simulink model "HinfController"  (R2024b)
settings: Solver=FixedStepDiscrete  StartTime=0.0  StopTime=Inf  FixedStep=0.001  RelTol=1e-3
model workspace (MAT data in the model file):
  robot : robotics.RigidBodyTree (value not decoded)
settings Model: Creator=sung  LastModifiedBy=sung
settings HardwareCC: ProdBitPerLong=64  ProdHWDeviceType=Intel->x86-64 (Linux 64)
settings RTWCC: GenCodeOnly=on  Toolchain=CMake

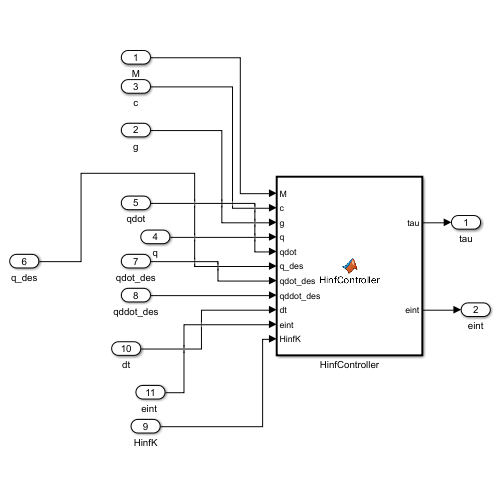
[thumbnail: Simulink's stored preview of the top-level diagram]
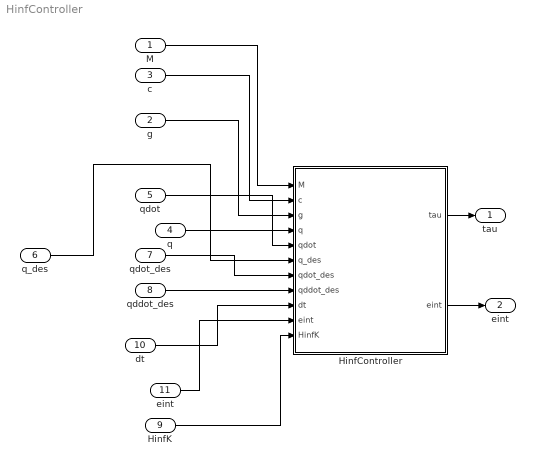
== system HinfController ==
  M : Inport  PortDimensions=[12,12]
  g : Inport  Port=2  PortDimensions=12
  c : Inport  Port=3  PortDimensions=12
  q : Inport  Port=4  PortDimensions=12
  qdot : Inport  Port=5  PortDimensions=12
  q_des : Inport  Port=6  PortDimensions=12
  qdot_des : Inport  Port=7  PortDimensions=12
  qddot_des : Inport  Port=8  PortDimensions=12
  HinfK : Inport  Port=9  PortDimensions=12
  dt : Inport  Port=10
  "eint " : Inport  Port=11
  HinfController : MATLAB Function  TreatAsAtomicUnit=on
  tau : Outport
  eint : Outport  Port=2
  wires:
  M/1 -> HinfController/1(M)
  qdot_des/1 -> HinfController/7(qdot_des)
  g/1 -> HinfController/3(g)
  c/1 -> HinfController/2(c)
  q/1 -> HinfController/4(q)
  qdot/1 -> HinfController/5(qdot)
  q_des/1 -> HinfController/6(q_des)
  qddot_des/1 -> HinfController/8(qddot_des)
  HinfController/1(tau) -> tau/1
  HinfController/2(eint) -> eint/1
  HinfK/1 -> HinfController/11(HinfK)
  dt/1 -> HinfController/9(dt)
  "eint "/1 -> HinfController/10("eint ")

== matlab function HinfController/HinfController ==
  data: M input size=[12,12]; tau output size=[12,1]; c input size=[12,1]; g input size=[12,1]; q input size=[12,1]; qdot input size=[12,1]; q_des input size=[12,1]; qdot_des input size=[12,1]; qddot_des input size=[12,1]; dt input; eint input size=[12,1]; HinfK input size=[12,1]; eint output
function [tau,eint]  = HinfController(M,c,g,q,qdot,q_des,qdot_des,qddot_des,dt,eint,HinfK)

e = q_des-q;
edot = qdot_des-qdot;
eint = eint+e.*dt;
qddot_ref =qddot_des+100*e+20*edot;

tau = M*qddot_ref+c+g+diag(HinfK)*(edot+20*e+100*eint);
